simulink model "LP_FxLMS"  (R2024b)
settings: Solver=FixedStepDiscrete  StartTime=0.0  StopTime=5  RelTol=1e-3
undefined symbols (not defined in the file): DiscIntNeverNeededParam, dspblkCoreblockFVToolHelper, gcbh
libraries: arduinolib x3, dspadpt3 x1
settings Model: DataTypeOverride=Off  MinMaxOverflowLogging=ForceOff  SimulationMode=accelerator  Creator=Administrator  LastModifiedBy=当幸福来敲门丶
settings DataIOCC: SaveOutput=off  SaveTime=off
settings OptimizationCC: BlockReduction=off  ConditionallyExecuteInputs=off  DefaultParameterBehavior=Inlined  InheritOutputTypeSmallerThanSingle=on  DefaultUnderspecifiedDataType=single
settings DebuggingCC: SignalRangeChecking=error  AlgebraicLoopMsg=error  ArtificialAlgebraicLoopMsg=error  SingleTaskRateTransMsg=error  IntegerOverflowMsg=none  ParameterDowncastMsg=none  ParameterOverflowMsg=none  ParameterPrecisionLossMsg=none  UnconnectedInputMsg=warning  UnconnectedOutputMsg=warning  UnconnectedLineMsg=warning  IntegerSaturationMsg=none
settings HardwareCC: ProdBitPerPointer=32  ProdBitPerSizeT=32  ProdBitPerPtrDiffT=32  ProdLargestAtomicFloat=None  ProdIntDivRoundTo=Undefined  ProdEndianess=Unspecified  ProdWordSize=32  ProdHWDeviceType=ASIC/FPGA->ASIC/FPGA  TargetBitPerPointer=64  TargetBitPerSizeT=64  TargetBitPerPtrDiffT=64  TargetLongLongMode=on  TargetIntDivRoundTo=Zero  TargetEndianess=LittleEndian  TargetWordSize=64  TargetHWDeviceType=Custom Processor->MATLAB Host Computer  ProdEqTarget=off

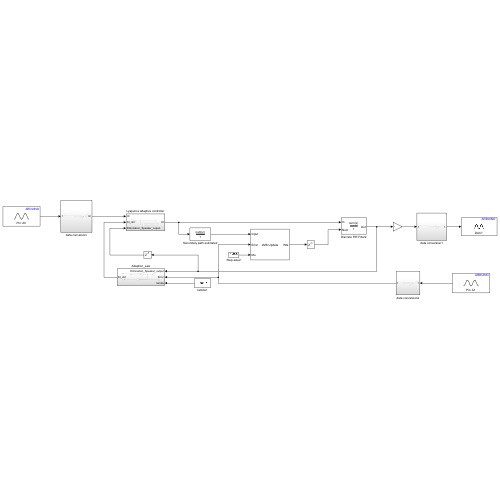
[thumbnail: Simulink's stored preview of the top-level diagram]
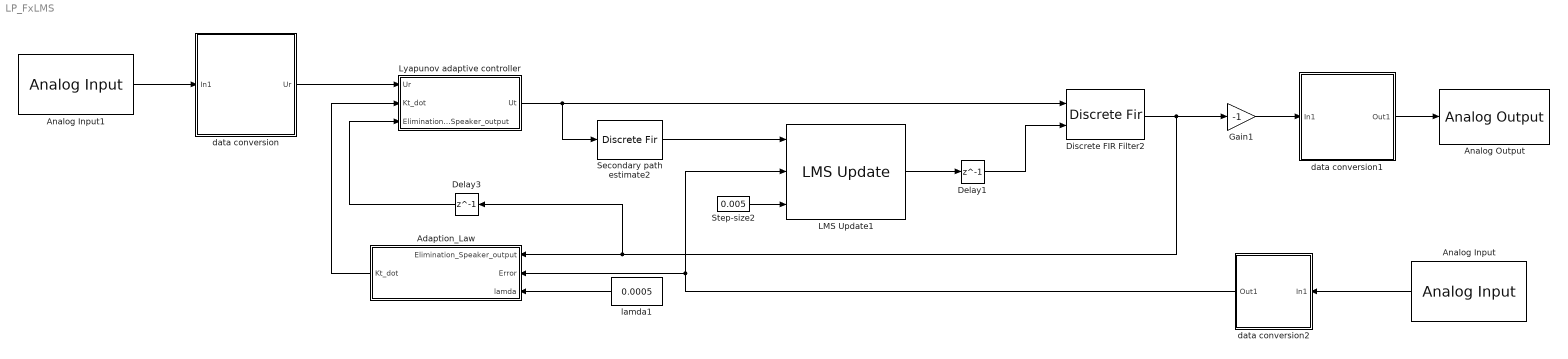
== system LP_FxLMS ==
  Adaption_Law : Subsystem
  Analog Input : arduinolib/Analog Input  pinNumber=1  ReadResultsOnly=off  ConversionTriggerSource=Software  ExternalTriggerType=uint32(0)  OutputDataType=uint16  EnableConversionCompleteNotify=off  EnableOuputStatus=off  SampleTime=1/8000  blockPlatform=arduino
      settings: SourceProductName=Common
  Analog Input1 : arduinolib/Analog Input  pinNumber=0  ReadResultsOnly=off  ConversionTriggerSource=Software  ExternalTriggerType=uint32(0)  OutputDataType=uint16  EnableConversionCompleteNotify=off  EnableOuputStatus=off  SampleTime=1/8000  blockPlatform=arduino
      settings: SourceProductName=Common
  Analog Output : arduinolib/Analog Output  blockPlatform=ARDUINO  DACpin=DAC1
      settings: SourceProductName=Common
  Delay1 : Delay  DelayLength=1
  Delay3 : Delay  DelayLength=1
  Discrete FIR Filter2 : DiscreteFir  CoefSource=Input port
      settings: InputPortMap=u0,u1
  Gain1 : Gain  Gain=-1
  LMS Update1 : dspadpt3/LMS Update  Method=LMS  Length=32  NumFilters=1  StepSizeSource=Input port  StepSize=0.1  LeakageFactor=1.0  InitialConditions=0  AdaptiveFilterMode=Tapped delay-line FIR filter  EnableAdaptInput=off  EnableResetInput=off  SimulateUsing=Interpreted execution
  Lyapunov adaptive controller : Subsystem
  Secondary path estimate2 : DiscreteFir  LoadFcn=dspblkCoreblockFVToolHelper(gcbh,'load');  Coefficients="[-0.2\t-0.20\t-0.08\t-0.41\t-0.05\t0.23\t0.19\t0.35\t0.13\t0.12\t0.05\t-0.36\t0.19\t0.07\t0.03\t0.29\t0.08\t0.11\t-0.08\t-0.05\t-0.08\t0.04\t0.07\t0.34\t-0.37\t0.02\t-0.22\t-0.04\t-0.12\t-0.10\t-0\t-0.15]"
      settings: CopyFcn=dspblkCoreblockFVToolHelper(gcbh,'copy');  DeleteFcn=dspblkCoreblockFVToolHelper(gcbh,'close');  ModelCloseFcn=dspblkCoreblockFVToolHelper(gcbh,'close');  PreSaveFcn=dspblkCoreblockFVToolHelper(gcbh,'presave');  PostSaveFcn=dspblkCoreblockFVToolHelper(gcbh,'postsave');  CloseFcn=dspblkCoreblockFVToolHelper(gcbh,'close');
  Step-size2 : Constant  Value=0.005  SampleTime=-1
  data conversion : Subsystem
  data conversion1 : Subsystem
  data conversion2 : Subsystem
  lamda1 : Constant  Value=0.0005  SampleTime=-1
  wires:
  Analog Input/1 -> data conversion2/1(In1)
  Analog Input1/1 -> data conversion/1(In1)
  data conversion1/1(Out1) -> Analog Output/1
  Discrete FIR Filter2/1 -> Gain1/1, Adaption_Law/1(Elimination_Speaker_output), Delay3/1
  Gain1/1 -> data conversion1/1(In1)
  Delay1/1 -> Discrete FIR Filter2/2
  Step-size2/1 -> LMS Update1/3
  LMS Update1/1 -> Delay1/1
  Delay3/1 -> Lyapunov adaptive controller/3(Elimination_Speaker_output)
  Lyapunov adaptive controller/1(Ut) -> Secondary path estimate2/1, Discrete FIR Filter2/1
  data conversion/1(Ur) -> Lyapunov adaptive controller/1(Ur)
  Adaption_Law/1(Kt_dot) -> Lyapunov adaptive controller/2(Kt_dot)
  data conversion2/1(Out1) -> Adaption_Law/2(Error), LMS Update1/2
  lamda1/1 -> Adaption_Law/3(lamda)
  Secondary path estimate2/1 -> LMS Update1/1

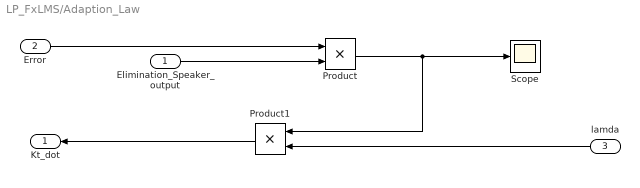
== system LP_FxLMS/Adaption_Law ==
  Elimination_Speaker_output : Inport
  Error : Inport  Port=2
  lamda : Inport  Port=3
  Product : Product
  Product1 : Product
  Scope : Scope
  Kt_dot : Outport
  wires:
  Product1/1 -> Kt_dot/1
  Elimination_Speaker_output/1 -> Product/2
  Error/1 -> Product/1
  Product/1 -> Product1/1, Scope/1
  lamda/1 -> Product1/2

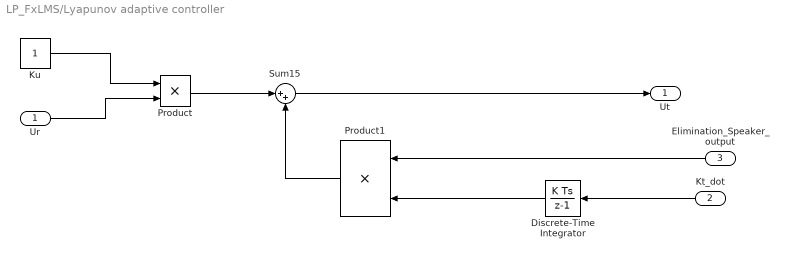
== system LP_FxLMS/Lyapunov adaptive controller ==
  Ur : Inport
  Kt_dot : Inport  Port=2
  Elimination_Speaker_output : Inport  Port=3
  Discrete-Time Integrator : DiscreteIntegrator  gainval=2  SampleTime=-1  ICPrevOutput=DiscIntNeverNeededParam  ICPrevScaledInput=DiscIntNeverNeededParam
  Ku : Constant
  Product : Product
  Product1 : Product
  Sum15 : Sum  Inputs=|++
  Ut : Outport
  wires:
  Elimination_Speaker_output/1 -> Product1/1
  Kt_dot/1 -> Discrete-Time Integrator/1
  Ur/1 -> Product/2
  Product1/1 -> Sum15/2
  Sum15/1 -> Ut/1
  Product/1 -> Sum15/1
  Discrete-Time Integrator/1 -> Product1/2
  Ku/1 -> Product/1

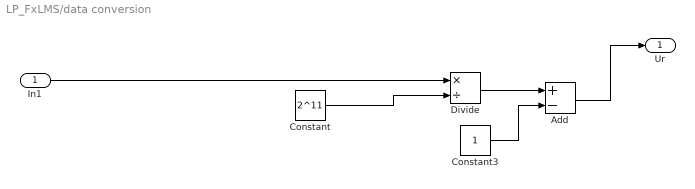
== system LP_FxLMS/data conversion ==
  In1 : Inport
  Add : Sum  Inputs=+-
  Constant : Constant  Value=2^11
  Constant3 : Constant
  Divide : Product  Inputs=*/
  Ur : Outport
  wires:
  Constant/1 -> Divide/2
  In1/1 -> Divide/1
  Divide/1 -> Add/1
  Constant3/1 -> Add/2
  Add/1 -> Ur/1

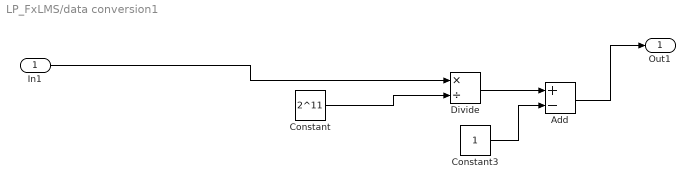
== system LP_FxLMS/data conversion1 ==
  In1 : Inport
  Add : Sum  Inputs=+-  OutDataTypeStr=uint16
  Constant : Constant  Value=2^11
  Constant3 : Constant
  Divide : Product  Inputs=*/
  Out1 : Outport
  wires:
  Constant/1 -> Divide/2
  In1/1 -> Divide/1
  Divide/1 -> Add/1
  Constant3/1 -> Add/2
  Add/1 -> Out1/1

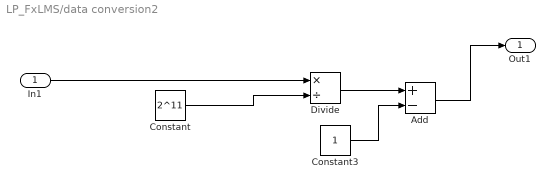
== system LP_FxLMS/data conversion2 ==
  In1 : Inport
  Add : Sum  Inputs=+-
  Constant : Constant  Value=2^11
  Constant3 : Constant
  Divide : Product  Inputs=*/
  Out1 : Outport
  wires:
  Constant/1 -> Divide/2
  In1/1 -> Divide/1
  Divide/1 -> Add/1
  Constant3/1 -> Add/2
  Add/1 -> Out1/1
